simulink model "dof3"  (R2019a)
settings: Solver=VariableStepAuto  StartTime=0.0  StopTime=10.0  RelTol=1e-3
values from neighbouring files (symbols this model uses):
  c1 = 2    [code.m]
  c2 = 2    [code.m]
  k1 = 2    [code.m]
  k2 = 2    [code.m]
  k3 = 2    [code.m]
  k4 = 2    [code.m]
  m1 = 1    [code.m]
  m2 = 1    [code.m]
  m3 = 1    [code.m]
settings Model: Creator=lenovo  LastModifiedBy=lenovo

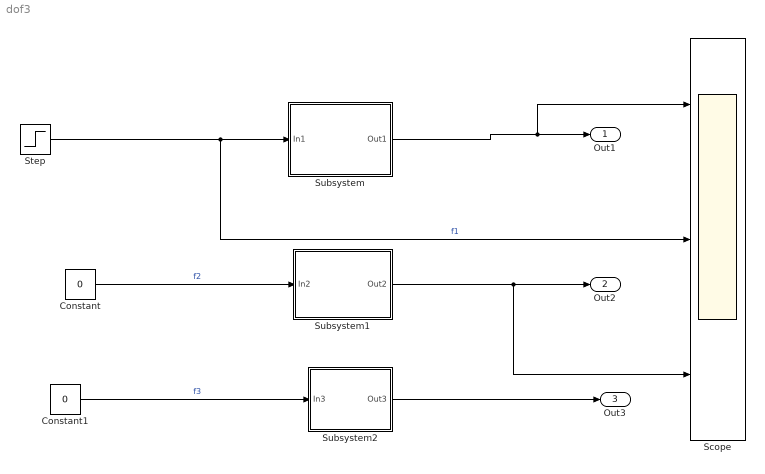
== system dof3 ==
  Constant : Constant  Value=0
  Constant1 : Constant  Value=0
  Scope : Scope  NumInputPorts=3
  Step : Step  SampleTime=0
  Subsystem : Subsystem
  Subsystem1 : Subsystem
  Subsystem2 : Subsystem
  Out1 : Outport
  Out2 : Outport  Port=2
  Out3 : Outport  Port=3
  wires:
  Step/1 -> Scope/2, Subsystem/1(In1)  "f1"
  Constant/1 -> Subsystem1/1(In2)  "f2"
  Subsystem1/1(Out2) -> Scope/3, Out2/1
  Constant1/1 -> Subsystem2/1(In3)  "f3"
  Subsystem2/1(Out3) -> Out3/1
  Subsystem/1(Out1) -> Scope/1, Out1/1

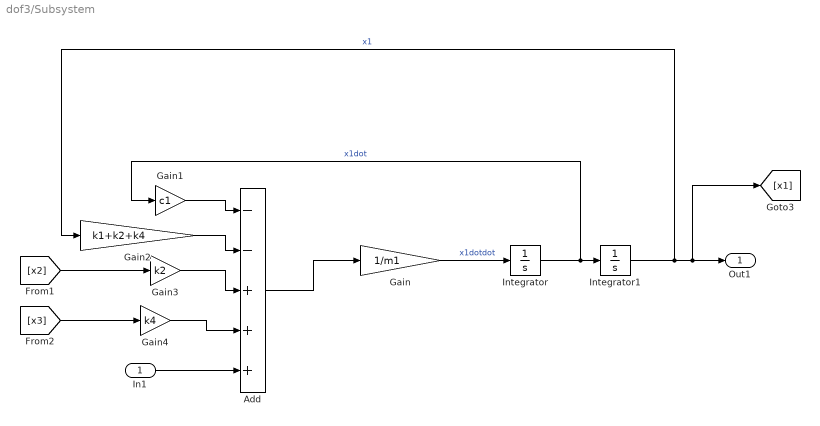
== system dof3/Subsystem ==
  In1 : Inport
  Add : Sum  Inputs=--+++
  Gain : Gain  Gain=1/m1
  Gain1 : Gain  Gain=c1
  Gain2 : Gain  Gain=k1+k2+k4
  Gain3 : Gain  Gain=k2
  Gain4 : Gain  Gain=k4
  Integrator : Integrator
  Integrator1 : Integrator
  Out1 : Outport
  wires:
  Integrator/1 -> Gain1/1, Integrator1/1  "x1dot"
  In1/1 -> Add/5
  Gain1/1 -> Add/1
  Gain3/1 -> Add/3
  [x3] -> Gain4/1
  Add/1 -> Gain/1
  [x2] -> Gain3/1
  Gain2/1 -> Add/2
  Integrator1/1 -> Gain2/1, Out1/1, [x1]  "x1"
  Gain4/1 -> Add/4
  Gain/1 -> Integrator/1  "x1dotdot"

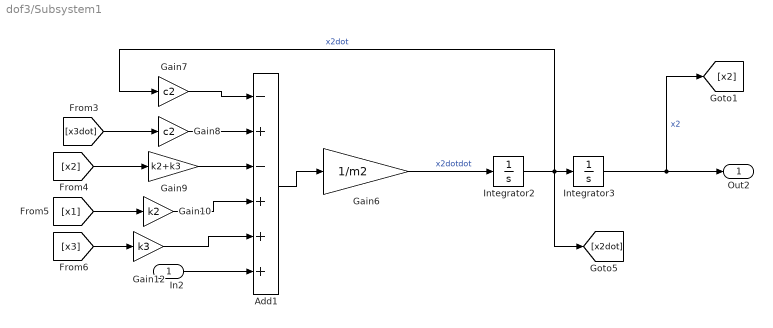
== system dof3/Subsystem1 ==
  In2 : Inport
  Add1 : Sum  Inputs=-+-+++
  Gain10 : Gain  Gain=k2
  Gain12 : Gain  Gain=k3
  Gain6 : Gain  Gain=1/m2
  Gain7 : Gain  Gain=c2
  Gain8 : Gain  Gain=c2
  Gain9 : Gain  Gain=k2+k3
  Integrator2 : Integrator
  Integrator3 : Integrator
  Out2 : Outport
  wires:
  [x2] -> Gain9/1
  Gain6/1 -> Integrator2/1  "x2dotdot"
  In2/1 -> Add1/6
  Gain8/1 -> Add1/2
  Integrator3/1 -> Out2/1, [x2]  "x2"
  Integrator2/1 -> [x2dot], Gain7/1, Integrator3/1  "x2dot"
  Gain9/1 -> Add1/3
  Add1/1 -> Gain6/1
  Gain7/1 -> Add1/1
  Gain10/1 -> Add1/4
  [x3dot] -> Gain8/1
  [x1] -> Gain10/1
  Gain12/1 -> Add1/5
  [x3] -> Gain12/1

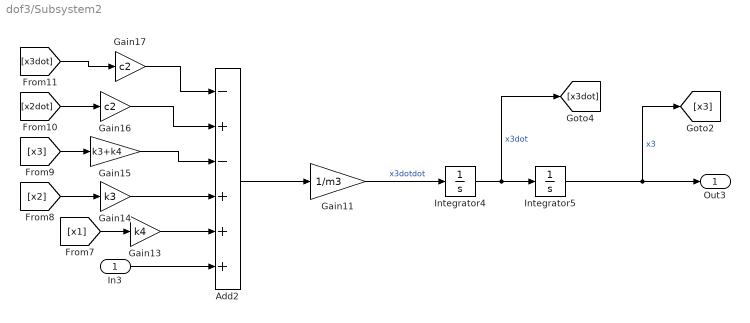
== system dof3/Subsystem2 ==
  In3 : Inport
  Add2 : Sum  Inputs=-+-+++
  Gain11 : Gain  Gain=1/m3
  Gain13 : Gain  Gain=k4
  Gain14 : Gain  Gain=k3
  Gain15 : Gain  Gain=k3+k4
  Gain16 : Gain  Gain=c2
  Gain17 : Gain  Gain=c2
  Integrator4 : Integrator
  Integrator5 : Integrator
  Out3 : Outport
  wires:
  Gain11/1 -> Integrator4/1  "x3dotdot"
  Integrator4/1 -> [x3dot], Integrator5/1  "x3dot"
  [x3dot] -> Gain17/1
  Gain13/1 -> Add2/5
  [x2] -> Gain14/1
  Gain15/1 -> Add2/3
  Gain17/1 -> Add2/1
  Gain14/1 -> Add2/4
  In3/1 -> Add2/6
  [x1] -> Gain13/1
  [x2dot] -> Gain16/1
  Gain16/1 -> Add2/2
  Integrator5/1 -> Out3/1, [x3]  "x3"
  Add2/1 -> Gain11/1
  [x3] -> Gain15/1
